simulink model "case8"  (R2024b)
settings: Solver=FixedStepAuto  StartTime=0  StopTime=1  FixedStep=1e-7  RelTol=1e-3
values from neighbouring files (symbols this model uses):
  SG_D_1_D = 0.01056    [IEEE9_case_parameters.m]    (also in case1_parameters.m; case2_parameters.m; case3_parameters.m; case4_parameters.m)
  SG_D_1_EnableSaturation = 0    [IEEE9_case_parameters.m]    (also in case1_parameters.m; case2_parameters.m; case3_parameters.m; case4_parameters.m)
  SG_D_1_f0 = 60    [IEEE9_case_parameters.m]    (also in case1_parameters.m; case2_parameters.m; case3_parameters.m; case4_parameters.m)
  SG_D_1_H = 7.5    [IEEE9_case_parameters.m]    (also in case1_parameters.m; case2_parameters.m; case3_parameters.m; case4_parameters.m)
  SG_D_1_K_A = 20    [IEEE9_case_parameters.m]    (also in case1_parameters.m; case2_parameters.m; case3_parameters.m; case4_parameters.m)
  SG_D_1_K_E = 1.000000e+1    (= 10)    [IEEE9_case_parameters.m]    (also in case1_parameters.m; case2_parameters.m; case3_parameters.m; case4_parameters.m)
  SG_D_1_K_F = 2.363    [IEEE9_case_parameters.m]    (also in case1_parameters.m; case2_parameters.m; case3_parameters.m; case4_parameters.m)
  SG_D_1_K_s = 0.5    [IEEE9_case_parameters.m]    (also in case1_parameters.m = 5; case2_parameters.m = 5; case3_parameters.m = 5; case4_parameters.m = 5)
  SG_D_1_R_a = 0.001088    [IEEE9_case_parameters.m]    (also in case1_parameters.m; case2_parameters.m; case3_parameters.m; case4_parameters.m)
  SG_D_1_S_A = 1    [IEEE9_case_parameters.m]    (also in case1_parameters.m; case2_parameters.m; case3_parameters.m; case4_parameters.m)
  SG_D_1_S_B = 0.103    [IEEE9_case_parameters.m]    (also in case1_parameters.m; case2_parameters.m; case3_parameters.m; case4_parameters.m)
  SG_D_1_S_N = 10.659857    [IEEE9_case_parameters.m]    (also in case1_parameters.m; case2_parameters.m; case3_parameters.m; case4_parameters.m)
  SG_D_1_SpeedPara = 200    [IEEE9_case_parameters.m]    (also in case1_parameters.m; case2_parameters.m; case3_parameters.m; case4_parameters.m)
  SG_D_1_T_0 = 0.720173    [IEEE9_case_parameters.m]    (also in case1_parameters.m = 0.755522; case2_parameters.m = 0.808931; case3_parameters.m = 0.869402; case4_parameters.m = 0.729316)
  SG_D_1_T_1 = 0.3    [IEEE9_case_parameters.m]    (also in case1_parameters.m; case2_parameters.m; case3_parameters.m; case4_parameters.m)
  SG_D_1_T_2 = 0.05    [IEEE9_case_parameters.m]    (also in case1_parameters.m; case2_parameters.m; case3_parameters.m; case4_parameters.m)
  SG_D_1_T_3 = 0.02    [IEEE9_case_parameters.m]    (also in case1_parameters.m; case2_parameters.m; case3_parameters.m; case4_parameters.m)
  SG_D_1_T_4 = 0.005    [IEEE9_case_parameters.m]    (also in case1_parameters.m; case2_parameters.m; case3_parameters.m; case4_parameters.m)
  SG_D_1_T_A = 0.02    [IEEE9_case_parameters.m]    (also in case1_parameters.m; case2_parameters.m; case3_parameters.m; case4_parameters.m)
  SG_D_1_T_dd = 8.000000e+0    (= 8)    [IEEE9_case_parameters.m]    (also in case1_parameters.m; case2_parameters.m; case3_parameters.m; case4_parameters.m)
  SG_D_1_T_ddd = 0.04    [IEEE9_case_parameters.m]    (also in case1_parameters.m; case2_parameters.m; case3_parameters.m; case4_parameters.m)
  SG_D_1_T_E = 0.314    [IEEE9_case_parameters.m]    (also in case1_parameters.m; case2_parameters.m; case3_parameters.m; case4_parameters.m)
  SG_D_1_T_F = 0.35    [IEEE9_case_parameters.m]    (also in case1_parameters.m; case2_parameters.m; case3_parameters.m; case4_parameters.m)
  SG_D_1_T_qd = 0.8    [IEEE9_case_parameters.m]    (also in case1_parameters.m; case2_parameters.m; case3_parameters.m; case4_parameters.m)
  SG_D_1_T_qdd = 0.02    [IEEE9_case_parameters.m]    (also in case1_parameters.m; case2_parameters.m; case3_parameters.m; case4_parameters.m)
  SG_D_1_T_speed = 0.1    [IEEE9_case_parameters.m]    (also in case1_parameters.m = 200; case2_parameters.m = 200; case3_parameters.m = 200; case4_parameters.m = 200)
  SG_D_1_T_w = 0.5    [IEEE9_case_parameters.m]    (also in case1_parameters.m; case2_parameters.m; case3_parameters.m; case4_parameters.m)
  SG_D_1_V_ref = 1.990276    [IEEE9_case_parameters.m]    (also in case1_parameters.m = 2.042296; case2_parameters.m = 2.051388; case3_parameters.m = 2.089584; case4_parameters.m = 2.01845)
  SG_D_1_w_ref = 376.991118    [IEEE9_case_parameters.m]    (also in case1_parameters.m; case2_parameters.m; case3_parameters.m; case4_parameters.m)
  SG_D_1_wb = 6.000000e+1    (= 60)    [IEEE9_case_parameters.m]    (also in case1_parameters.m; case2_parameters.m; case3_parameters.m; case4_parameters.m)
  SG_D_1_x_d = 1.9    [IEEE9_case_parameters.m]    (also in case1_parameters.m; case2_parameters.m; case3_parameters.m; case4_parameters.m)
  SG_D_1_x_dd = 0.302    [IEEE9_case_parameters.m]    (also in case1_parameters.m; case2_parameters.m; case3_parameters.m; case4_parameters.m)
  SG_D_1_x_ddd = 0.204    [IEEE9_case_parameters.m]    (also in case1_parameters.m; case2_parameters.m; case3_parameters.m; case4_parameters.m)
  SG_D_1_x_l = 0.05    [IEEE9_case_parameters.m]    (also in case1_parameters.m; case2_parameters.m; case3_parameters.m; case4_parameters.m)
  SG_D_1_x_q = 1.3    [IEEE9_case_parameters.m]    (also in case1_parameters.m; case2_parameters.m; case3_parameters.m; case4_parameters.m)
  SG_D_1_x_qd = 0.5    [IEEE9_case_parameters.m]    (also in case1_parameters.m; case2_parameters.m; case3_parameters.m; case4_parameters.m)
  SG_D_1_x_qdd = 0.3    [IEEE9_case_parameters.m]    (also in case1_parameters.m; case2_parameters.m; case3_parameters.m; case4_parameters.m)
  SG_D_2_D = 0.02    [IEEE9_case_parameters.m]    (also in case1_parameters.m; case2_parameters.m; case3_parameters.m; case4_parameters.m)
  SG_D_2_EnableSaturation = 0    [IEEE9_case_parameters.m]    (also in case1_parameters.m; case2_parameters.m; case3_parameters.m; case4_parameters.m)
  SG_D_2_f0 = 60    [IEEE9_case_parameters.m]    (also in case1_parameters.m; case2_parameters.m; case3_parameters.m; case4_parameters.m)
  SG_D_2_H = 8.000000e+0    (= 8)    [IEEE9_case_parameters.m]    (also in case1_parameters.m; case2_parameters.m; case3_parameters.m; case4_parameters.m)
  SG_D_2_K_A = 20    [IEEE9_case_parameters.m]    (also in case1_parameters.m; case2_parameters.m; case3_parameters.m; case4_parameters.m)
  SG_D_2_K_E = 1.000000e+1    (= 10)    [IEEE9_case_parameters.m]    (also in case1_parameters.m; case2_parameters.m; case3_parameters.m; case4_parameters.m)
  SG_D_2_K_F = 2.363    [IEEE9_case_parameters.m]    (also in case1_parameters.m; case2_parameters.m; case3_parameters.m; case4_parameters.m)
  SG_D_2_K_s = 0.5    [IEEE9_case_parameters.m]    (also in case1_parameters.m = 4; case2_parameters.m = 4; case3_parameters.m = 4; case4_parameters.m = 4)
  SG_D_2_R_a = 0.001088    [IEEE9_case_parameters.m]    (also in case1_parameters.m; case2_parameters.m; case3_parameters.m; case4_parameters.m)
  SG_D_2_S_A = 1    [IEEE9_case_parameters.m]    (also in case1_parameters.m; case2_parameters.m; case3_parameters.m; case4_parameters.m)
  SG_D_2_S_B = 0.103    [IEEE9_case_parameters.m]    (also in case1_parameters.m; case2_parameters.m; case3_parameters.m; case4_parameters.m)
  SG_D_2_S_N = 10.659857    [IEEE9_case_parameters.m]    (also in case1_parameters.m; case2_parameters.m; case3_parameters.m; case4_parameters.m)
  SG_D_2_SpeedPara = 200    [IEEE9_case_parameters.m]    (also in case1_parameters.m; case2_parameters.m; case3_parameters.m; case4_parameters.m)
  SG_D_2_T_0 = 1.632913    [IEEE9_case_parameters.m]    (also in case1_parameters.m = 1.632925; case2_parameters.m = 1.632915; case3_parameters.m = 1.632914; case4_parameters.m = 1.632927)
  SG_D_2_T_1 = 0.2    [IEEE9_case_parameters.m]    (also in case1_parameters.m; case2_parameters.m; case3_parameters.m; case4_parameters.m)
  SG_D_2_T_2 = 0.05    [IEEE9_case_parameters.m]    (also in case1_parameters.m; case2_parameters.m; case3_parameters.m; case4_parameters.m)
  SG_D_2_T_3 = 0.02    [IEEE9_case_parameters.m]    (also in case1_parameters.m; case2_parameters.m; case3_parameters.m; case4_parameters.m)
  SG_D_2_T_4 = 0.005    [IEEE9_case_parameters.m]    (also in case1_parameters.m; case2_parameters.m; case3_parameters.m; case4_parameters.m)
  SG_D_2_T_A = 0.02    [IEEE9_case_parameters.m]    (also in case1_parameters.m; case2_parameters.m; case3_parameters.m; case4_parameters.m)
  SG_D_2_T_dd = 7.9    [IEEE9_case_parameters.m]    (also in case1_parameters.m; case2_parameters.m; case3_parameters.m; case4_parameters.m)
  SG_D_2_T_ddd = 0.04    [IEEE9_case_parameters.m]    (also in case1_parameters.m; case2_parameters.m; case3_parameters.m; case4_parameters.m)
  SG_D_2_T_E = 0.314    [IEEE9_case_parameters.m]    (also in case1_parameters.m; case2_parameters.m; case3_parameters.m; case4_parameters.m)
  SG_D_2_T_F = 0.35    [IEEE9_case_parameters.m]    (also in case1_parameters.m; case2_parameters.m; case3_parameters.m; case4_parameters.m)
  SG_D_2_T_qd = 0.8    [IEEE9_case_parameters.m]    (also in case1_parameters.m; case2_parameters.m; case3_parameters.m; case4_parameters.m)
  SG_D_2_T_qdd = 0.015    [IEEE9_case_parameters.m]    (also in case1_parameters.m; case2_parameters.m; case3_parameters.m; case4_parameters.m)
  SG_D_2_T_speed = 0.1    [IEEE9_case_parameters.m]    (also in case1_parameters.m = 150; case2_parameters.m = 150; case3_parameters.m = 150; case4_parameters.m = 150)
  SG_D_2_T_w = 0.35    [IEEE9_case_parameters.m]    (also in case1_parameters.m; case2_parameters.m; case3_parameters.m; case4_parameters.m)
  SG_D_2_V_ref = 2.58547    [IEEE9_case_parameters.m]    (also in case1_parameters.m = 2.597896; case2_parameters.m = 2.587136; case3_parameters.m = 2.586042; case4_parameters.m = 2.599679)
  SG_D_2_w_ref = 376.991118    [IEEE9_case_parameters.m]    (also in case1_parameters.m; case2_parameters.m; case3_parameters.m; case4_parameters.m)
  SG_D_2_wb = 6.000000e+1    (= 60)    [IEEE9_case_parameters.m]    (also in case1_parameters.m; case2_parameters.m; case3_parameters.m; case4_parameters.m)
  SG_D_2_x_d = 1.8    [IEEE9_case_parameters.m]    (also in case1_parameters.m; case2_parameters.m; case3_parameters.m; case4_parameters.m)
  SG_D_2_x_dd = 0.302    [IEEE9_case_parameters.m]    (also in case1_parameters.m; case2_parameters.m; case3_parameters.m; case4_parameters.m)
  SG_D_2_x_ddd = 0.204    [IEEE9_case_parameters.m]    (also in case1_parameters.m; case2_parameters.m; case3_parameters.m; case4_parameters.m)
  SG_D_2_x_l = 0.05    [IEEE9_case_parameters.m]    (also in case1_parameters.m; case2_parameters.m; case3_parameters.m; case4_parameters.m)
  SG_D_2_x_q = 1.25    [IEEE9_case_parameters.m]    (also in case1_parameters.m; case2_parameters.m; case3_parameters.m; case4_parameters.m)
  SG_D_2_x_qd = 0.5    [IEEE9_case_parameters.m]    (also in case1_parameters.m; case2_parameters.m; case3_parameters.m; case4_parameters.m)
  SG_D_2_x_qdd = 0.3    [IEEE9_case_parameters.m]    (also in case1_parameters.m; case2_parameters.m; case3_parameters.m; case4_parameters.m)
  SG_D_3_D = 0.02    [IEEE9_case_parameters.m]    (also in case1_parameters.m; case2_parameters.m; case3_parameters.m; case4_parameters.m)
  SG_D_3_EnableSaturation = 0    [IEEE9_case_parameters.m]    (also in case1_parameters.m; case2_parameters.m; case3_parameters.m; case4_parameters.m)
  SG_D_3_f0 = 60    [IEEE9_case_parameters.m]    (also in case1_parameters.m; case2_parameters.m; case3_parameters.m; case4_parameters.m)
  SG_D_3_H = 7.7    [IEEE9_case_parameters.m]    (also in case1_parameters.m; case2_parameters.m; case3_parameters.m; case4_parameters.m)
  SG_D_3_K_A = 20    [IEEE9_case_parameters.m]    (also in case1_parameters.m; case2_parameters.m; case3_parameters.m; case4_parameters.m)
  SG_D_3_K_E = 1.000000e+1    (= 10)    [IEEE9_case_parameters.m]    (also in case1_parameters.m; case2_parameters.m; case3_parameters.m; case4_parameters.m)
  SG_D_3_K_F = 2.363    [IEEE9_case_parameters.m]    (also in case1_parameters.m; case2_parameters.m; case3_parameters.m; case4_parameters.m)
  SG_D_3_K_s = 0.2    [IEEE9_case_parameters.m]    (also in case1_parameters.m = 2; case2_parameters.m = 2; case3_parameters.m = 2; case4_parameters.m = 2)
  SG_D_3_R_a = 0.001088    [IEEE9_case_parameters.m]    (also in case1_parameters.m; case2_parameters.m; case3_parameters.m; case4_parameters.m)
  SG_D_3_S_A = 1    [IEEE9_case_parameters.m]    (also in case1_parameters.m; case2_parameters.m; case3_parameters.m; case4_parameters.m)
  SG_D_3_S_B = 0.103    [IEEE9_case_parameters.m]    (also in case1_parameters.m; case2_parameters.m; case3_parameters.m; case4_parameters.m)
  SG_D_3_S_N = 10.659857    [IEEE9_case_parameters.m]    (also in case1_parameters.m; case2_parameters.m; case3_parameters.m; case4_parameters.m)
  SG_D_3_SpeedPara = 200    [IEEE9_case_parameters.m]    (also in case1_parameters.m; case2_parameters.m; case3_parameters.m; case4_parameters.m)
  SG_D_3_T_0 = 0.850788    [IEEE9_case_parameters.m]    (also in case1_parameters.m = 0.850786; case2_parameters.m = 0.850787; case3_parameters.m; case4_parameters.m = 0.850786)
  SG_D_3_T_1 = 0.2    [IEEE9_case_parameters.m]    (also in case1_parameters.m; case2_parameters.m; case3_parameters.m; case4_parameters.m)
  SG_D_3_T_2 = 0.05    [IEEE9_case_parameters.m]    (also in case1_parameters.m; case2_parameters.m; case3_parameters.m; case4_parameters.m)
  SG_D_3_T_3 = 0.02    [IEEE9_case_parameters.m]    (also in case1_parameters.m; case2_parameters.m; case3_parameters.m; case4_parameters.m)
  SG_D_3_T_4 = 0.005    [IEEE9_case_parameters.m]    (also in case1_parameters.m; case2_parameters.m; case3_parameters.m; case4_parameters.m)
  SG_D_3_T_A = 0.02    [IEEE9_case_parameters.m]    (also in case1_parameters.m; case2_parameters.m; case3_parameters.m; case4_parameters.m)
  SG_D_3_T_dd = 8.1    [IEEE9_case_parameters.m]    (also in case1_parameters.m; case2_parameters.m; case3_parameters.m; case4_parameters.m)
  SG_D_3_T_ddd = 0.04    [IEEE9_case_parameters.m]    (also in case1_parameters.m; case2_parameters.m; case3_parameters.m; case4_parameters.m)
  SG_D_3_T_E = 0.314    [IEEE9_case_parameters.m]    (also in case1_parameters.m; case2_parameters.m; case3_parameters.m; case4_parameters.m)
  SG_D_3_T_F = 0.35    [IEEE9_case_parameters.m]    (also in case1_parameters.m; case2_parameters.m; case3_parameters.m; case4_parameters.m)
  SG_D_3_T_qd = 0.8    [IEEE9_case_parameters.m]    (also in case1_parameters.m; case2_parameters.m; case3_parameters.m; case4_parameters.m)
  SG_D_3_T_qdd = 0.015    [IEEE9_case_parameters.m]    (also in case1_parameters.m; case2_parameters.m; case3_parameters.m; case4_parameters.m)
  SG_D_3_T_speed = 0.1    [IEEE9_case_parameters.m]    (also in case1_parameters.m = 180; case2_parameters.m = 180; case3_parameters.m = 180; case4_parameters.m = 180)
  SG_D_3_T_w = 0.4    [IEEE9_case_parameters.m]    (also in case1_parameters.m; case2_parameters.m; case3_parameters.m; case4_parameters.m)
  SG_D_3_V_ref = 1.892727    [IEEE9_case_parameters.m]    (also in case1_parameters.m = 1.906439; case2_parameters.m = 1.895535; case3_parameters.m = 1.892105; case4_parameters.m = 1.906598)
  SG_D_3_w_ref = 376.991118    [IEEE9_case_parameters.m]    (also in case1_parameters.m; case2_parameters.m; case3_parameters.m; case4_parameters.m)
  SG_D_3_wb = 6.000000e+1    (= 60)    [IEEE9_case_parameters.m]    (also in case1_parameters.m; case2_parameters.m; case3_parameters.m; case4_parameters.m)
  SG_D_3_x_d = 1.85    [IEEE9_case_parameters.m]    (also in case1_parameters.m; case2_parameters.m; case3_parameters.m; case4_parameters.m)
  SG_D_3_x_dd = 0.302    [IEEE9_case_parameters.m]    (also in case1_parameters.m; case2_parameters.m; case3_parameters.m; case4_parameters.m)
  SG_D_3_x_ddd = 0.204    [IEEE9_case_parameters.m]    (also in case1_parameters.m; case2_parameters.m; case3_parameters.m; case4_parameters.m)
  SG_D_3_x_l = 0.05    [IEEE9_case_parameters.m]    (also in case1_parameters.m; case2_parameters.m; case3_parameters.m; case4_parameters.m)
  SG_D_3_x_q = 1.2    [IEEE9_case_parameters.m]    (also in case1_parameters.m; case2_parameters.m; case3_parameters.m; case4_parameters.m)
  SG_D_3_x_qd = 0.5    [IEEE9_case_parameters.m]    (also in case1_parameters.m; case2_parameters.m; case3_parameters.m; case4_parameters.m)
  SG_D_3_x_qdd = 0.3    [IEEE9_case_parameters.m]    (also in case1_parameters.m; case2_parameters.m; case3_parameters.m; case4_parameters.m)
(part 7 of 12)

== system case8/SG_D_2/T_e_SG_D_2_block ==
  note: T_e_SG_D_2 in case8
      | $-\frac{\psi _{d,\mathrm{SG},D,2}\,\left(\psi _{q,\mathrm{SG},D,2}+\frac{\psi _{\mathrm{gq},\mathrm{SG},D,2}\,\left(x_{l}-x_{\mathrm{qdd}}\right)}{x_{l}-x_{\mathrm{qd}}}+\frac{\psi _{\mathrm{kq},\mathrm{SG},D,2}\,\left(x_{\mathrm{qd}}-x_{\mathrm{qdd}}\right)}{x_{l}-x_{\mathrm{qd}}}\right)}{x_{\mathrm{qdd}}}-\frac{\psi _{q,\mathrm{SG},D,2}\,\left(\frac{\psi _{\mathrm{1d},\mathrm{SG},D,2}\,\left(x_{\mathrm{dd}}-x_{\mathrm{ddd}}\right)}{x_{\mathrm{dd}}-x_{l}}-\psi _{d,\mathrm{SG},D,2}+\frac{\psi _{\mathrm{fd},\mathrm{SG},D,2}\,\left(x_{\mathrm{ddd}}-x_{l}\right)}{x_{\mathrm{dd}}-x_{l}}\right)}{x_{\mathrm{ddd}}}$
      | Automatically generated on 2025-10-31 19:30:01 .
  State_psi_d_SG_D_2_f5fd7 : Inport
  State_psi_gq_SG_D_2_6b895 : Inport  Port=2
  State_psi_kq_SG_D_2_20085 : Inport  Port=3
  State_psi_q_SG_D_2_d1f35 : Inport  Port=4
  State_psi_q_SG_D_2_dcfde : Inport  Port=5
  State_psi_1d_SG_D_2_b2612 : Inport  Port=6
  State_psi_d_SG_D_2_0c163 : Inport  Port=7
  State_psi_fd_SG_D_2_89a99 : Inport  Port=8
  Add_136e4 : Sum
  Add_53914 : Sum
  Add_61d82 : Sum
  Add_773d3 : Sum
  Add_83d4e : Sum
  Add_d6d3e : Sum
  Constant_-1_009c4 : Constant  Value=-1
  Constant_-1_892f0 : Constant  Value=-1
  Constant_-1_8f9af : Constant  Value=-1
  Constant_-1_ac596 : Constant  Value=-1
  Constant_-1_f984b : Constant  Value=-1
  Constant_x_dd_539a3 : Constant  Value=x_dd
  Constant_x_dd_5f008 : Constant  Value=x_dd
  Constant_x_dd_6f2fd : Constant  Value=x_dd
  Constant_x_ddd_43beb : Constant  Value=x_ddd
  Constant_x_ddd_5974d : Constant  Value=x_ddd
  Constant_x_ddd_df5c6 : Constant  Value=x_ddd
  Constant_x_l_1b4ed : Constant  Value=x_l
  Constant_x_l_21d9c : Constant  Value=x_l
  Constant_x_l_82116 : Constant  Value=x_l
  Constant_x_l_9e257 : Constant  Value=x_l
  Constant_x_l_ccf6e : Constant  Value=x_l
  Constant_x_l_da74a : Constant  Value=x_l
  Constant_x_qd_305c8 : Constant  Value=x_qd
  Constant_x_qd_c568d : Constant  Value=x_qd
  Constant_x_qd_e5ab0 : Constant  Value=x_qd
  Constant_x_qdd_23062 : Constant  Value=x_qdd
  Constant_x_qdd_642dc : Constant  Value=x_qdd
  Constant_x_qdd_bb207 : Constant  Value=x_qdd
  Divide_1324e : Product  Inputs=*/
  Divide_1c984 : Product  Inputs=*/
  Divide_4d64c : Product  Inputs=*/
  Divide_4f496 : Product  Inputs=*/
  Divide_cc898 : Product  Inputs=*/
  Divide_d40a1 : Product  Inputs=*/
  Product_2226e : Product
  Product_299f3 : Product
  Product_47b76 : Product
  Product_50440 : Product
  Product_582c1 : Product
  Product_6692e : Product
  Product_6acbc : Product
  Product_6f7a7 : Product
  Product_75582 : Product
  Product_78bca : Product
  Product_7dbfb : Product
  Subtract_00826 : Sum  Inputs=+-
  Subtract_1342e : Sum  Inputs=+-
  Subtract_3f03d : Sum  Inputs=+-
  Subtract_5a401 : Sum  Inputs=+-
  Subtract_9aa6a : Sum  Inputs=+-
  Subtract_c14d6 : Sum  Inputs=+-
  Subtract_caa32 : Sum  Inputs=+-
  Blockout_T_e_SG_D_2_37eed : Outport
  wires:
  Constant_-1_892f0/1 -> Product_299f3/1
  Divide_1c984/1 -> Subtract_3f03d/1
  Constant_-1_ac596/1 -> Product_2226e/1
  Constant_x_l_da74a/1 -> Product_2226e/2
  Constant_x_qd_e5ab0/1 -> Subtract_caa32/1
  Product_78bca/1 -> Divide_1c984/1
  Product_2226e/1 -> Add_773d3/1
  Divide_cc898/1 -> Subtract_c14d6/2
  Constant_x_qdd_642dc/1 -> Subtract_caa32/2
  Constant_x_qdd_23062/1 -> Divide_4f496/2
  Constant_x_ddd_5974d/1 -> Subtract_9aa6a/2
  Constant_x_qdd_bb207/1 -> Add_773d3/2
  Constant_x_l_82116/1 -> Product_299f3/2
  Constant_-1_009c4/1 -> Product_75582/1
  Constant_x_l_ccf6e/1 -> Product_75582/2
  Constant_-1_8f9af/1 -> Product_6acbc/1
  State_psi_1d_SG_D_2_b2612/1 -> Product_6acbc/2
  Constant_x_dd_5f008/1 -> Subtract_9aa6a/1
  Divide_4d64c/1 -> Subtract_3f03d/2
  State_psi_gq_SG_D_2_6b895/1 -> Product_78bca/1
  Add_773d3/1 -> Product_78bca/2
  Subtract_3f03d/1 -> Add_136e4/1
  Constant_x_dd_539a3/1 -> Subtract_00826/1
  Product_299f3/1 -> Add_83d4e/1
  Product_582c1/1 -> Product_50440/1
  Constant_x_qd_305c8/1 -> Add_83d4e/2
  State_psi_kq_SG_D_2_20085/1 -> Product_6692e/1
  Subtract_caa32/1 -> Product_6692e/2
  Product_75582/1 -> Add_61d82/1
  State_psi_q_SG_D_2_dcfde/1 -> Product_47b76/1
  Constant_x_qd_c568d/1 -> Add_61d82/2
  Product_6acbc/1 -> Product_6f7a7/1
  Divide_1324e/1 -> Add_53914/2
  Subtract_9aa6a/1 -> Product_6f7a7/2
  Constant_x_l_1b4ed/1 -> Subtract_00826/2
  Constant_x_ddd_df5c6/1 -> Subtract_5a401/1
  Constant_x_dd_6f2fd/1 -> Subtract_1342e/1
  Constant_x_l_21d9c/1 -> Subtract_5a401/2
  Add_53914/1 -> Blockout_T_e_SG_D_2_37eed/1
  Add_83d4e/1 -> Divide_1c984/2
  Product_6692e/1 -> Divide_4d64c/1
  Product_50440/1 -> Divide_4f496/1
  State_psi_d_SG_D_2_f5fd7/1 -> Product_582c1/2
  Add_61d82/1 -> Divide_4d64c/2
  Product_6f7a7/1 -> Divide_d40a1/1
  Subtract_00826/1 -> Divide_d40a1/2
  Constant_x_l_9e257/1 -> Subtract_1342e/2
  State_psi_fd_SG_D_2_89a99/1 -> Product_7dbfb/1
  Constant_x_ddd_43beb/1 -> Divide_1324e/2
  Product_47b76/1 -> Divide_1324e/1
  Subtract_5a401/1 -> Product_7dbfb/2
  Divide_d40a1/1 -> Add_d6d3e/1
  State_psi_d_SG_D_2_0c163/1 -> Add_d6d3e/2
  Add_d6d3e/1 -> Subtract_c14d6/1
  Product_7dbfb/1 -> Divide_cc898/1
  Subtract_1342e/1 -> Divide_cc898/2
  Constant_-1_f984b/1 -> Product_582c1/1
  State_psi_q_SG_D_2_d1f35/1 -> Add_136e4/2
  Add_136e4/1 -> Product_50440/2
  Subtract_c14d6/1 -> Product_47b76/2
  Divide_4f496/1 -> Add_53914/1

== system case8/SG_D_2/d_E_fd_SG_D_2_block ==
  note: d_E_fd_SG_D_2 in case8
      | $\frac{V_{f,\mathrm{SG},D,2}-E_{\mathrm{fd},\mathrm{SG},D,2}\,K_{E}}{T_{E}}$
      | Automatically generated on 2025-10-31 19:29:56 .
  State_E_fd_SG_D_2_423a9 : Inport
  State_V_f_SG_D_2_b3f2e : Inport  Port=2
  Add_25b17 : Sum
  Constant_-1_61e25 : Constant  Value=-1
  Constant_K_E_4608d : Constant  Value=K_E
  Constant_T_E_94d73 : Constant  Value=T_E
  Divide_83db9 : Product  Inputs=*/
  Product_0c2eb : Product
  Product_b81d0 : Product
  Blockout_d_E_fd_SG_D_2_a4411 : Outport
  wires:
  Constant_-1_61e25/1 -> Product_0c2eb/1
  State_E_fd_SG_D_2_423a9/1 -> Product_0c2eb/2
  Product_0c2eb/1 -> Product_b81d0/1
  Constant_K_E_4608d/1 -> Product_b81d0/2
  Product_b81d0/1 -> Add_25b17/1
  Constant_T_E_94d73/1 -> Divide_83db9/2
  State_V_f_SG_D_2_b3f2e/1 -> Add_25b17/2
  Add_25b17/1 -> Divide_83db9/1
  Divide_83db9/1 -> Blockout_d_E_fd_SG_D_2_a4411/1

== system case8/SG_D_2/d_Px_1_SG_D_2_block ==
  note: d_Px_1_SG_D_2 in case8
      | $\frac{w_{\mathrm{SG},D,2}-2\,\pi \,f_{0}}{T_{w}}-\frac{\mathrm{Px}_{1,\mathrm{SG},D,2}}{T_{w}}$
      | Automatically generated on 2025-10-31 19:29:57 .
  State_Px_1_SG_D_2_1fdac : Inport
  State_w_SG_D_2_e8896 : Inport  Port=2
  Add_4c732 : Sum
  Add_5193f : Sum
  Constant_-1_69875 : Constant  Value=-1
  Constant_-2.0_497bd : Constant  Value=-2.0
  Constant_T_w_ca876 : Constant  Value=T_w
  Constant_T_w_db7d6 : Constant  Value=T_w
  Constant_f0_826e2 : Constant  Value=f0
  Constant_pi_6538e : Constant  Value=pi
  Divide_c5870 : Product  Inputs=*/
  Divide_dfdb0 : Product  Inputs=*/
  Product_c48f8 : Product
  Product_d32d8 : Product
  Product_f4819 : Product
  Blockout_d_Px_1_SG_D_2_3d98f : Outport
  wires:
  Constant_-2.0_497bd/1 -> Product_d32d8/1
  State_w_SG_D_2_e8896/1 -> Add_5193f/2
  Constant_pi_6538e/1 -> Product_d32d8/2
  Product_d32d8/1 -> Product_c48f8/1
  Constant_f0_826e2/1 -> Product_c48f8/2
  Constant_-1_69875/1 -> Product_f4819/1
  State_Px_1_SG_D_2_1fdac/1 -> Product_f4819/2
  Product_c48f8/1 -> Add_5193f/1
  Product_f4819/1 -> Divide_dfdb0/1
  Constant_T_w_ca876/1 -> Divide_dfdb0/2
  Add_5193f/1 -> Divide_c5870/1
  Constant_T_w_db7d6/1 -> Divide_c5870/2
  Divide_dfdb0/1 -> Add_4c732/1
  Divide_c5870/1 -> Add_4c732/2
  Add_4c732/1 -> Blockout_d_Px_1_SG_D_2_3d98f/1

== system case8/SG_D_2/d_Px_2_SG_D_2_block ==
  note: d_Px_2_SG_D_2 in case8
      | $\frac{\mathrm{Px}_{1,\mathrm{SG},D,2}-T_{2}\,\left(\frac{\mathrm{Px}_{1,\mathrm{SG},D,2}}{T_{w}}-\frac{w_{\mathrm{SG},D,2}-2\,\pi \,f_{0}}{T_{w}}\right)}{T_{1}}-\frac{\mathrm{Px}_{2,\mathrm{SG},D,2}}{T_{1}}$
      | Automatically generated on 2025-10-31 19:29:57 .
  State_Px_2_SG_D_2_8f0fc : Inport
  State_Px_1_SG_D_2_d6347 : Inport  Port=2
  State_Px_1_SG_D_2_2790d : Inport  Port=3
  State_w_SG_D_2_770a4 : Inport  Port=4
  Add_36fde : Sum
  Add_9a15f : Sum
  Add_aade0 : Sum
  Add_f8e8c : Sum
  Constant_-1_a4b81 : Constant  Value=-1
  Constant_-1_c1136 : Constant  Value=-1
  Constant_-2.0_37c36 : Constant  Value=-2.0
  Constant_T_1_313c9 : Constant  Value=T_1
  Constant_T_1_99444 : Constant  Value=T_1
  Constant_T_2_214de : Constant  Value=T_2
  Constant_T_w_0eda0 : Constant  Value=T_w
  Constant_T_w_a5a3c : Constant  Value=T_w
  Constant_f0_de17b : Constant  Value=f0
  Constant_pi_860d9 : Constant  Value=pi
  Divide_48f92 : Product  Inputs=*/
  Divide_8705a : Product  Inputs=*/
  Divide_c60fc : Product  Inputs=*/
  Divide_fd14b : Product  Inputs=*/
  Product_30601 : Product
  Product_5dbb0 : Product
  Product_6c663 : Product
  Product_bcc78 : Product
  Product_e83f9 : Product
  Blockout_d_Px_2_SG_D_2_834a7 : Outport
  wires:
  Constant_-1_a4b81/1 -> Product_bcc78/1
  Constant_-2.0_37c36/1 -> Product_5dbb0/1
  Product_e83f9/1 -> Add_f8e8c/2
  State_w_SG_D_2_770a4/1 -> Add_aade0/2
  Constant_pi_860d9/1 -> Product_5dbb0/2
  Product_5dbb0/1 -> Product_6c663/1
  State_Px_1_SG_D_2_2790d/1 -> Product_30601/2
  Constant_f0_de17b/1 -> Product_6c663/2
  State_Px_2_SG_D_2_8f0fc/1 -> Product_bcc78/2
  Constant_-1_c1136/1 -> Product_30601/1
  Product_6c663/1 -> Add_aade0/1
  Product_30601/1 -> Divide_48f92/1
  Constant_T_w_a5a3c/1 -> Divide_48f92/2
  Add_aade0/1 -> Divide_fd14b/1
  Constant_T_w_0eda0/1 -> Divide_fd14b/2
  Divide_48f92/1 -> Add_9a15f/1
  Divide_fd14b/1 -> Add_9a15f/2
  Constant_T_2_214de/1 -> Product_e83f9/1
  Add_9a15f/1 -> Product_e83f9/2
  State_Px_1_SG_D_2_d6347/1 -> Add_f8e8c/1
  Product_bcc78/1 -> Divide_c60fc/1
  Constant_T_1_99444/1 -> Divide_c60fc/2
  Add_f8e8c/1 -> Divide_8705a/1
  Constant_T_1_313c9/1 -> Divide_8705a/2
  Divide_c60fc/1 -> Add_36fde/1
  Divide_8705a/1 -> Add_36fde/2
  Add_36fde/1 -> Blockout_d_Px_2_SG_D_2_834a7/1

== system case8/SG_D_2/d_Px_3_SG_D_2_block ==
  note: d_Px_3_SG_D_2 in case8
      | $\frac{\mathrm{Px}_{2,\mathrm{SG},D,2}+T_{4}\,\left(\frac{\mathrm{Px}_{1,\mathrm{SG},D,2}-T_{2}\,\left(\frac{\mathrm{Px}_{1,\mathrm{SG},D,2}}{T_{w}}-\frac{w_{\mathrm{SG},D,2}-2\,\pi \,f_{0}}{T_{w}}\right)}{T_{1}}-\frac{\mathrm{Px}_{2,\mathrm{SG},D,2}}{T_{1}}\right)}{T_{3}}-\frac{\mathrm{Px}_{3,\mathrm{SG},D,2}}{T_{3}}$
      | Automatically generated on 2025-10-31 19:29:58 .
  State_Px_3_SG_D_2_a00f9 : Inport
  State_Px_2_SG_D_2_e8830 : Inport  Port=2
  State_Px_2_SG_D_2_b92ad : Inport  Port=3
  State_Px_1_SG_D_2_7fb84 : Inport  Port=4
  State_Px_1_SG_D_2_3fef0 : Inport  Port=5
  State_w_SG_D_2_e0f2c : Inport  Port=6
  Add_3c5a4 : Sum
  Add_45cb1 : Sum
  Add_478fb : Sum
  Add_98fbb : Sum
  Add_c2473 : Sum
  Add_e28b8 : Sum
  Constant_-1_3360d : Constant  Value=-1
  Constant_-1_357f0 : Constant  Value=-1
  Constant_-1_d3ba9 : Constant  Value=-1
  Constant_-2.0_0c54b : Constant  Value=-2.0
  Constant_T_1_5ca23 : Constant  Value=T_1
  Constant_T_1_645ff : Constant  Value=T_1
  Constant_T_2_9f8bc : Constant  Value=T_2
  Constant_T_3_25afd : Constant  Value=T_3
  Constant_T_3_a1775 : Constant  Value=T_3
  Constant_T_4_97e42 : Constant  Value=T_4
  Constant_T_w_3102e : Constant  Value=T_w
  Constant_T_w_b16aa : Constant  Value=T_w
  Constant_f0_93310 : Constant  Value=f0
  Constant_pi_9ec7e : Constant  Value=pi
  Divide_03af6 : Product  Inputs=*/
  Divide_5d724 : Product  Inputs=*/
  Divide_70b54 : Product  Inputs=*/
  Divide_cf44f : Product  Inputs=*/
  Divide_d5d88 : Product  Inputs=*/
  Divide_fecd8 : Product  Inputs=*/
  Product_0c09d : Product
  Product_1e5b6 : Product
  Product_83b7e : Product
  Product_87485 : Product
  Product_905df : Product
  Product_be3e8 : Product
  Product_df649 : Product
  Blockout_d_Px_3_SG_D_2_f4998 : Outport
  wires:
  Constant_-2.0_0c54b/1 -> Product_87485/1
  State_w_SG_D_2_e0f2c/1 -> Add_3c5a4/2
  Add_c2473/1 -> Divide_cf44f/1
  Constant_pi_9ec7e/1 -> Product_87485/2
  Constant_-1_d3ba9/1 -> Product_be3e8/1
  Product_87485/1 -> Product_83b7e/1
  State_Px_2_SG_D_2_b92ad/1 -> Product_be3e8/2
  State_Px_1_SG_D_2_3fef0/1 -> Product_905df/2
  Divide_cf44f/1 -> Add_478fb/2
  Constant_f0_93310/1 -> Product_83b7e/2
  Constant_-1_357f0/1 -> Product_905df/1
  Product_83b7e/1 -> Add_3c5a4/1
  Product_905df/1 -> Divide_d5d88/1
  Constant_T_w_b16aa/1 -> Divide_d5d88/2
  Divide_70b54/1 -> Add_478fb/1
  Add_3c5a4/1 -> Divide_03af6/1
  Product_0c09d/1 -> Add_98fbb/2
  Constant_T_w_3102e/1 -> Divide_03af6/2
  Divide_d5d88/1 -> Add_45cb1/1
  State_Px_1_SG_D_2_7fb84/1 -> Add_98fbb/1
  Divide_03af6/1 -> Add_45cb1/2
  Constant_-1_3360d/1 -> Product_1e5b6/1
  Constant_T_2_9f8bc/1 -> Product_0c09d/1
  Add_45cb1/1 -> Product_0c09d/2
  Product_be3e8/1 -> Divide_fecd8/1
  Constant_T_1_645ff/1 -> Divide_fecd8/2
  Add_98fbb/1 -> Divide_5d724/1
  Constant_T_1_5ca23/1 -> Divide_5d724/2
  Divide_fecd8/1 -> Add_e28b8/1
  Divide_5d724/1 -> Add_e28b8/2
  Constant_T_4_97e42/1 -> Product_df649/1
  Add_e28b8/1 -> Product_df649/2
  State_Px_3_SG_D_2_a00f9/1 -> Product_1e5b6/2
  State_Px_2_SG_D_2_e8830/1 -> Add_c2473/1
  Product_df649/1 -> Add_c2473/2
  Product_1e5b6/1 -> Divide_70b54/1
  Constant_T_3_a1775/1 -> Divide_70b54/2
  Constant_T_3_25afd/1 -> Divide_cf44f/2
  Add_478fb/1 -> Blockout_d_Px_3_SG_D_2_f4998/1

== system case8/SG_D_2/d_R_f_SG_D_2_block ==
  note: d_R_f_SG_D_2 in case8
      | $-\frac{R_{f,\mathrm{SG},D,2}-\frac{E_{\mathrm{fd},\mathrm{SG},D,2}\,K_{F}}{T_{F}}}{T_{F}}$
      | Automatically generated on 2025-10-31 19:29:56 .
  State_E_fd_SG_D_2_59077 : Inport
  State_R_f_SG_D_2_76268 : Inport  Port=2
  Constant_K_F_8fb42 : Constant  Value=K_F
  Constant_T_F_492c7 : Constant  Value=T_F
  Constant_T_F_7a55d : Constant  Value=T_F
  Divide_1705c : Product  Inputs=*/
  Divide_c19ba : Product  Inputs=*/
  Product_2540e : Product
  Subtract_aa317 : Sum  Inputs=+-
  Blockout_d_R_f_SG_D_2_8501b : Outport
  wires:
  Constant_T_F_7a55d/1 -> Divide_1705c/2
  State_E_fd_SG_D_2_59077/1 -> Product_2540e/1
  Constant_K_F_8fb42/1 -> Product_2540e/2
  State_R_f_SG_D_2_76268/1 -> Subtract_aa317/2
  Product_2540e/1 -> Divide_1705c/1
  Divide_1705c/1 -> Subtract_aa317/1
  Constant_T_F_492c7/1 -> Divide_c19ba/2
  Subtract_aa317/1 -> Divide_c19ba/1
  Divide_c19ba/1 -> Blockout_d_R_f_SG_D_2_8501b/1

== system case8/SG_D_2/d_T_m_SG_D_2_block ==
  note: d_T_m_SG_D_2 in case8
      | $-\frac{T_{m,\mathrm{SG},D,2}-T_{0}+\frac{\mathrm{SpeedPara}\,\left(w_{\mathrm{SG},D,2}-w_{\mathrm{ref}}\right)}{2\,f_{0}\,\pi }}{T_{\mathrm{speed}}}$
      | Automatically generated on 2025-10-31 19:29:54 .
  State_w_SG_D_2_f6fcd : Inport
  State_T_m_SG_D_2_95b0e : Inport  Port=2
  Add_2317b : Sum
  Add_41ec9 : Sum
  Constant_-1_4ba95 : Constant  Value=-1
  Constant_2.0_25eb2 : Constant  Value=2.0
  Constant_SpeedPara_0fd14 : Constant  Value=SpeedPara
  Constant_T_0_72408 : Constant  Value=T_0
  Constant_T_speed_db217 : Constant  Value=T_speed
  Constant_f0_1dd2e : Constant  Value=f0
  Constant_pi_74fbc : Constant  Value=pi
  Constant_w_ref_3c240 : Constant  Value=w_ref
  Divide_b7933 : Product  Inputs=*/
  Divide_e5622 : Product  Inputs=*/
  Product_35d20 : Product
  Product_815ed : Product
  Product_d1949 : Product
  Product_f5924 : Product
  Subtract_c4e7f : Sum  Inputs=+-
  Blockout_d_T_m_SG_D_2_9d432 : Outport
  wires:
  Constant_pi_74fbc/1 -> Product_f5924/2
  Constant_-1_4ba95/1 -> Product_815ed/1
  Constant_w_ref_3c240/1 -> Add_2317b/2
  State_w_SG_D_2_f6fcd/1 -> Product_815ed/2
  Product_815ed/1 -> Add_2317b/1
  Add_41ec9/1 -> Subtract_c4e7f/1
  Add_2317b/1 -> Product_35d20/2
  Constant_2.0_25eb2/1 -> Product_f5924/1
  Constant_SpeedPara_0fd14/1 -> Product_35d20/1
  Product_f5924/1 -> Product_d1949/1
  Constant_f0_1dd2e/1 -> Product_d1949/2
  Product_35d20/1 -> Divide_b7933/1
  Product_d1949/1 -> Divide_b7933/2
  Divide_b7933/1 -> Add_41ec9/1
  Constant_T_0_72408/1 -> Add_41ec9/2
  State_T_m_SG_D_2_95b0e/1 -> Subtract_c4e7f/2
  Subtract_c4e7f/1 -> Divide_e5622/1
  Constant_T_speed_db217/1 -> Divide_e5622/2
  Divide_e5622/1 -> Blockout_d_T_m_SG_D_2_9d432/1

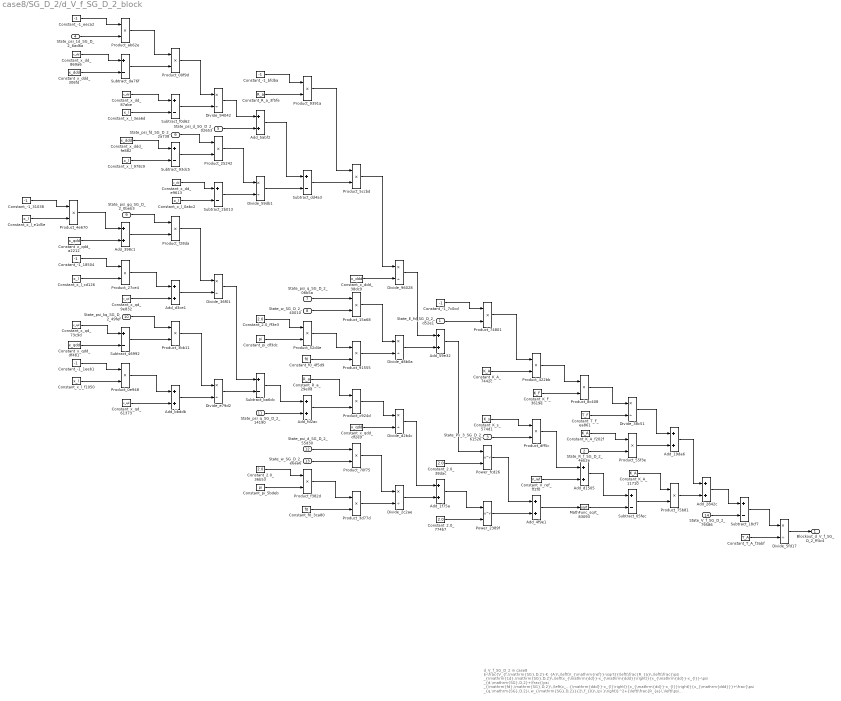
== system case8/SG_D_2/d_V_f_SG_D_2_block ==
  note: d_V_f_SG_D_2 in case8
      | $-\frac{V_{f,\mathrm{SG},D,2}-K_{A}\,\left(V_{\mathrm{ref}}-\sqrt{{\left(\frac{R_{a}\,\left(\frac{\psi _{\mathrm{1d},\mathrm{SG},D,2}\,\left(x_{\mathrm{dd}}-x_{\mathrm{ddd}}\right)}{x_{\mathrm{dd}}-x_{l}}-\psi _{d,\mathrm{SG},D,2}+\frac{\psi _{\mathrm{fd},\mathrm{SG},D,2}\,\left(x_{\mathrm{ddd}}-x_{l}\right)}{x_{\mathrm{dd}}-x_{l}}\right)}{x_{\mathrm{ddd}}}+\frac{\psi _{q,\mathrm{SG},D,2}\,w_{\mathrm{SG},D,2}}{2\,f_{0}\,\pi }\right)}^2+{\left(\frac{R_{a}\,\left(\psi _{q,\mathrm{SG},D,2}+\frac{\psi _{\mathrm{gq},\mathrm{SG},D,2}\,\left(x_{l}-x_{\mathrm{qdd}}\right)}{x_{l}-x_{\mathrm{qd}}}+\frac{\psi _{\mathrm{kq},\mathrm{SG},D,2}\,\left(x_{\mathrm{qd}}-x_{\mathrm{qdd}}\right)}{x_{l}-x_{\mathrm{qd}}}\right)}{x_{\mathrm{qdd}}}+\frac{\psi _{d,\mathrm{SG},D,2}\,w_{\mathrm{SG},D,2}}{2\,f_{0}\,\pi }\right)}^2}+K_{s}\,\mathrm{Px}_{3,\mathrm{SG},D,2}\right)-K_{A}\,R_{f,\mathrm{SG},D,2}+\frac{E_{\mathrm{fd},\mathrm{SG},D,2}\,K_{A}\,K_{F}}{T_{F}}}{T_{A}}$
      | Automatically generated on 2025-10-31 19:29:55 .
  State_E_fd_SG_D_2_d52e1 : Inport
  State_R_f_SG_D_2_4eb2e : Inport  Port=2
  State_Px_3_SG_D_2_61526 : Inport  Port=3
  State_psi_1d_SG_D_2_6ad6a : Inport  Port=4
  State_psi_d_SG_D_2_02653 : Inport  Port=5
  State_psi_fd_SG_D_2_2a738 : Inport  Port=6
  State_psi_q_SG_D_2_06b5a : Inport  Port=7
  State_w_SG_D_2_40010 : Inport  Port=8
  State_psi_gq_SG_D_2_0beb3 : Inport  Port=9
  State_psi_kq_SG_D_2_49fef : Inport  Port=10
  State_psi_q_SG_D_2_14190 : Inport  Port=11
  State_psi_d_SG_D_2_55d30 : Inport  Port=12
  State_w_SG_D_2_e6aa6 : Inport  Port=13
  State_V_f_SG_D_2_79586 : Inport  Port=14
  Add_19da6 : Sum
  Add_1f75a : Sum
  Add_2842c : Sum
  Add_398c1 : Sum
  Add_4f9e1 : Sum
  Add_59e32 : Sum
  Add_5abf2 : Sum
  Add_bbddb : Sum
  Add_d1505 : Sum
  Add_d3ce1 : Sum
  Add_fd2ac : Sum
  Constant_-1_18504 : Constant  Value=-1
  Constant_-1_1eeb1 : Constant  Value=-1
  Constant_-1_31038 : Constant  Value=-1
  Constant_-1_7c0cd : Constant  Value=-1
  Constant_-1_bfdba : Constant  Value=-1
  Constant_-1_eeca2 : Constant  Value=-1
  Constant_2.0_36b53 : Constant  Value=2.0
  Constant_2.0_38dac : Constant  Value=2.0
  Constant_2.0_774b7 : Constant  Value=2.0
  Constant_2.0_ff3e3 : Constant  Value=2.0
  Constant_K_A_11710 : Constant  Value=K_A
  Constant_K_A_7442c : Constant  Value=K_A
  Constant_K_A_f202f : Constant  Value=K_A
  Constant_K_F_3619e : Constant  Value=K_F
  Constant_K_s_574d1 : Constant  Value=K_s
  Constant_R_a_29e0d : Constant  Value=R_a
  Constant_R_a_3f5fe : Constant  Value=R_a
  Constant_T_A_f3abf : Constant  Value=T_A
  Constant_T_F_ea861 : Constant  Value=T_F
  Constant_V_ref_ff2f0 : Constant  Value=V_ref
  Constant_f0_3ca80 : Constant  Value=f0
  Constant_f0_4f5d9 : Constant  Value=f0
  Constant_pi_5bdeb : Constant  Value=pi
  Constant_pi_df3dc : Constant  Value=pi
  Constant_x_dd_869a6 : Constant  Value=x_dd
  Constant_x_dd_87abe : Constant  Value=x_dd
  Constant_x_dd_e9613 : Constant  Value=x_dd
  Constant_x_ddd_306fd : Constant  Value=x_ddd
  Constant_x_ddd_38dc9 : Constant  Value=x_ddd
  Constant_x_ddd_fe882 : Constant  Value=x_ddd
  Constant_x_l_0abc2 : Constant  Value=x_l
  Constant_x_l_3ea6d : Constant  Value=x_l
  Constant_x_l_978c9 : Constant  Value=x_l
  Constant_x_l_cd126 : Constant  Value=x_l
  Constant_x_l_e1d5e : Constant  Value=x_l
  Constant_x_l_f1050 : Constant  Value=x_l
  Constant_x_qd_61373 : Constant  Value=x_qd
  Constant_x_qd_73c9d : Constant  Value=x_qd
  Constant_x_qd_9e832 : Constant  Value=x_qd
  Constant_x_qdd_a2212 : Constant  Value=x_qdd
  Constant_x_qdd_df2e9 : Constant  Value=x_qdd
  Constant_x_qdd_df4b1 : Constant  Value=x_qdd
  Divide_2c2ae : Product  Inputs=*/
  Divide_36f01 : Product  Inputs=*/
  Divide_38c51 : Product  Inputs=*/
  Divide_59db1 : Product  Inputs=*/
  Divide_5fd17 : Product  Inputs=*/
  Divide_94042 : Product  Inputs=*/
  Divide_96028 : Product  Inputs=*/
  Divide_d2b4c : Product  Inputs=*/
  Divide_d8b0a : Product  Inputs=*/
  Divide_e79d2 : Product  Inputs=*/
  MathFunc_sqrt_83093 : Sqrt
  Power_2389f : Math  Operator=pow
  Power_fcd26 : Math  Operator=pow
  Product_00f9d : Product
  Product_0e948 : Product
  Product_15a68 : Product
  Product_25242 : Product
  Product_27ce4 : Product
  Product_3bb11 : Product
  Product_3d77d : Product
  Product_422bb : Product
  Product_4e670 : Product
  Product_52d4e : Product
  Product_55f3e : Product
  Product_5ccbd : Product
  Product_70f75 : Product
  Product_74801 : Product
  Product_75b81 : Product
  Product_8c408 : Product
  Product_91555 : Product
  Product_9391a : Product
  Product_ab62e : Product
  Product_c924d : Product
  Product_dff5c : Product
  Product_f28da : Product
  Product_f382d : Product
  Subtract_05fec : Sum  Inputs=+-
  Subtract_18cf7 : Sum  Inputs=+-
  Subtract_2b013 : Sum  Inputs=+-
  Subtract_46992 : Sum  Inputs=+-
  Subtract_93dc5 : Sum  Inputs=+-
  Subtract_ba6cb : Sum  Inputs=+-
  Subtract_da76f : Sum  Inputs=+-
  Subtract_dd4a3 : Sum  Inputs=+-
  Subtract_f0d62 : Sum  Inputs=+-
  Blockout_d_V_f_SG_D_2_ff4c4 : Outport
  wires:
  Constant_-1_eeca2/1 -> Product_ab62e/1
  Constant_2.0_ff3e3/1 -> Product_52d4e/1
  Constant_-1_31038/1 -> Product_4e670/1
  Product_52d4e/1 -> Product_91555/1
  Product_4e670/1 -> Add_398c1/1
  Constant_x_l_f1050/1 -> Product_0e948/2
  Constant_x_l_e1d5e/1 -> Product_4e670/2
  State_psi_1d_SG_D_2_6ad6a/1 -> Product_ab62e/2
  Constant_x_l_0abc2/1 -> Subtract_2b013/2
  Constant_x_dd_869a6/1 -> Subtract_da76f/1
  Product_c924d/1 -> Divide_d2b4c/1
  Constant_x_ddd_306fd/1 -> Subtract_da76f/2
  Constant_x_qd_61373/1 -> Add_bbddb/2
  Add_398c1/1 -> Product_f28da/2
  Constant_x_qdd_a2212/1 -> Add_398c1/2
  Constant_-1_18504/1 -> Product_27ce4/1
  Constant_x_dd_e9613/1 -> Subtract_2b013/1
  Subtract_ba6cb/1 -> Add_fd2ac/1
  Power_fcd26/1 -> Add_4f9e1/1
  Constant_x_l_cd126/1 -> Product_27ce4/2
  Constant_2.0_36b53/1 -> Product_f382d/1
  Constant_x_qd_73c9d/1 -> Subtract_46992/1
  Constant_pi_5bdeb/1 -> Product_f382d/2
  Subtract_dd4a3/1 -> Product_5ccbd/2
  Constant_x_qdd_df4b1/1 -> Subtract_46992/2
  State_psi_fd_SG_D_2_2a738/1 -> Product_25242/1
  Constant_-1_1eeb1/1 -> Product_0e948/1
  Product_ab62e/1 -> Product_00f9d/1
  State_w_SG_D_2_e6aa6/1 -> Product_70f75/2
  Subtract_da76f/1 -> Product_00f9d/2
  Constant_x_dd_87abe/1 -> Subtract_f0d62/1
  State_psi_q_SG_D_2_14190/1 -> Add_fd2ac/2
  State_w_SG_D_2_40010/1 -> Product_15a68/2
  Subtract_93dc5/1 -> Product_25242/2
  Constant_x_l_3ea6d/1 -> Subtract_f0d62/2
  Add_19da6/1 -> Add_2842c/1
  Constant_x_ddd_fe882/1 -> Subtract_93dc5/1
  Constant_x_l_978c9/1 -> Subtract_93dc5/2
  State_psi_gq_SG_D_2_0beb3/1 -> Product_f28da/1
  Product_27ce4/1 -> Add_d3ce1/1
  Subtract_2b013/1 -> Divide_59db1/2
  Constant_x_qd_9e832/1 -> Add_d3ce1/2
  Product_15a68/1 -> Divide_d8b0a/1
  State_psi_kq_SG_D_2_49fef/1 -> Product_3bb11/1
  Subtract_46992/1 -> Product_3bb11/2
  Product_25242/1 -> Divide_59db1/1
  State_V_f_SG_D_2_79586/1 -> Subtract_18cf7/2
  Product_0e948/1 -> Add_bbddb/1
  Product_00f9d/1 -> Divide_94042/1
  Divide_36f01/1 -> Subtract_ba6cb/1
  Subtract_f0d62/1 -> Divide_94042/2
  Product_f28da/1 -> Divide_36f01/1
  Add_d3ce1/1 -> Divide_36f01/2
  Product_3bb11/1 -> Divide_e79d2/1
  Divide_59db1/1 -> Subtract_dd4a3/2
  Constant_f0_4f5d9/1 -> Product_91555/2
  Add_bbddb/1 -> Divide_e79d2/2
  Divide_94042/1 -> Add_5abf2/1
  State_psi_d_SG_D_2_02653/1 -> Add_5abf2/2
  Divide_e79d2/1 -> Subtract_ba6cb/2
  Constant_-1_bfdba/1 -> Product_9391a/1
  Constant_R_a_3f5fe/1 -> Product_9391a/2
  Constant_f0_3ca80/1 -> Product_3d77d/2
  Add_5abf2/1 -> Subtract_dd4a3/1
  Product_9391a/1 -> Product_5ccbd/1
  Constant_pi_df3dc/1 -> Product_52d4e/2
  State_psi_q_SG_D_2_06b5a/1 -> Product_15a68/1
  Constant_R_a_29e0d/1 -> Product_c924d/1
  State_E_fd_SG_D_2_d52e1/1 -> Product_74801/2
  Add_fd2ac/1 -> Product_c924d/2
  State_psi_d_SG_D_2_55d30/1 -> Product_70f75/1
  Product_f382d/1 -> Product_3d77d/1
  Product_5ccbd/1 -> Divide_96028/1
  Constant_x_ddd_38dc9/1 -> Divide_96028/2
  Product_91555/1 -> Divide_d8b0a/2
  Constant_x_qdd_df2e9/1 -> Divide_d2b4c/2
  Product_70f75/1 -> Divide_2c2ae/1
  Product_3d77d/1 -> Divide_2c2ae/2
  Divide_96028/1 -> Add_59e32/1
  Divide_d8b0a/1 -> Add_59e32/2
  Divide_d2b4c/1 -> Add_1f75a/1
  Divide_2c2ae/1 -> Add_1f75a/2
  Constant_-1_7c0cd/1 -> Product_74801/1
  Add_59e32/1 -> Power_fcd26/1
  Constant_2.0_38dac/1 -> Power_fcd26/2
  Add_1f75a/1 -> Power_2389f/1
  Constant_2.0_774b7/1 -> Power_2389f/2
  Product_74801/1 -> Product_422bb/1
  Constant_K_A_7442c/1 -> Product_422bb/2
  Constant_K_s_574d1/1 -> Product_dff5c/1
  State_Px_3_SG_D_2_61526/1 -> Product_dff5c/2
  Power_2389f/1 -> Add_4f9e1/2
  Product_422bb/1 -> Product_8c408/1
  Constant_K_F_3619e/1 -> Product_8c408/2
  Product_dff5c/1 -> Add_d1505/1
  Constant_V_ref_ff2f0/1 -> Add_d1505/2
  Add_4f9e1/1 -> MathFunc_sqrt_83093/1
  Product_8c408/1 -> Divide_38c51/1
  Constant_T_F_ea861/1 -> Divide_38c51/2
  Constant_K_A_f202f/1 -> Product_55f3e/1
  State_R_f_SG_D_2_4eb2e/1 -> Product_55f3e/2
  Add_d1505/1 -> Subtract_05fec/1
  MathFunc_sqrt_83093/1 -> Subtract_05fec/2
  Divide_38c51/1 -> Add_19da6/1
  Product_55f3e/1 -> Add_19da6/2
  Constant_K_A_11710/1 -> Product_75b81/1
  Subtract_05fec/1 -> Product_75b81/2
  Product_75b81/1 -> Add_2842c/2
  Add_2842c/1 -> Subtract_18cf7/1
  Subtract_18cf7/1 -> Divide_5fd17/1
  Constant_T_A_f3abf/1 -> Divide_5fd17/2
  Divide_5fd17/1 -> Blockout_d_V_f_SG_D_2_ff4c4/1

== system case8/SG_D_2/d_psi_1d_SG_D_2_block ==
  note: d_psi_1d_SG_D_2 in case8
      | $-\frac{\psi _{\mathrm{1d},\mathrm{SG},D,2}-\psi _{\mathrm{fd},\mathrm{SG},D,2}+\frac{\left(x_{\mathrm{dd}}-x_{l}\right)\,\left(\frac{\psi _{\mathrm{1d},\mathrm{SG},D,2}\,\left(x_{\mathrm{dd}}-x_{\mathrm{ddd}}\right)}{x_{\mathrm{dd}}-x_{l}}-\psi _{d,\mathrm{SG},D,2}+\frac{\psi _{\mathrm{fd},\mathrm{SG},D,2}\,\left(x_{\mathrm{ddd}}-x_{l}\right)}{x_{\mathrm{dd}}-x_{l}}\right)}{x_{\mathrm{ddd}}}}{T_{\mathrm{ddd}}}$
      | Automatically generated on 2025-10-31 19:29:49 .
  State_psi_1d_SG_D_2_34802 : Inport
  State_psi_fd_SG_D_2_ceb12 : Inport  Port=2
  State_psi_1d_SG_D_2_f87fc : Inport  Port=3
  State_psi_d_SG_D_2_bd43f : Inport  Port=4
  State_psi_fd_SG_D_2_a1da1 : Inport  Port=5
  Add_02fd9 : Sum
  Add_58768 : Sum
  Add_caef2 : Sum
  Constant_-1_cc89f : Constant  Value=-1
  Constant_-1_de763 : Constant  Value=-1
  Constant_T_ddd_2034a : Constant  Value=T_ddd
  Constant_x_dd_0b947 : Constant  Value=x_dd
  Constant_x_dd_658ff : Constant  Value=x_dd
  Constant_x_dd_6b4c2 : Constant  Value=x_dd
  Constant_x_dd_def58 : Constant  Value=x_dd
  Constant_x_ddd_562a6 : Constant  Value=x_ddd
  Constant_x_ddd_5a3ac : Constant  Value=x_ddd
  Constant_x_ddd_97772 : Constant  Value=x_ddd
  Constant_x_l_1f432 : Constant  Value=x_l
  Constant_x_l_3d73c : Constant  Value=x_l
  Constant_x_l_79b40 : Constant  Value=x_l
  Constant_x_l_96b43 : Constant  Value=x_l
  Divide_56795 : Product  Inputs=*/
  Divide_84823 : Product  Inputs=*/
  Divide_b80b9 : Product  Inputs=*/
  Divide_be9cb : Product  Inputs=*/
  Product_22e0e : Product
  Product_53626 : Product
  Product_626ee : Product
  Product_6ef09 : Product
  Product_d49a0 : Product
  Subtract_0f8c3 : Sum  Inputs=+-
  Subtract_2f66b : Sum  Inputs=+-
  Subtract_62adb : Sum  Inputs=+-
  Subtract_9b5c5 : Sum  Inputs=+-
  Subtract_a35ae : Sum  Inputs=+-
  Subtract_b153c : Sum  Inputs=+-
  Blockout_d_psi_1d_SG_D_2_8d877 : Outport
  wires:
  Subtract_62adb/1 -> Product_6ef09/2
  Constant_x_l_96b43/1 -> Subtract_9b5c5/2
  Divide_be9cb/1 -> Add_02fd9/2
  Subtract_a35ae/1 -> Product_22e0e/2
  Constant_-1_cc89f/1 -> Product_53626/1
  Constant_x_dd_0b947/1 -> Subtract_b153c/1
  Divide_b80b9/1 -> Blockout_d_psi_1d_SG_D_2_8d877/1
  State_psi_fd_SG_D_2_ceb12/1 -> Add_58768/2
  State_psi_1d_SG_D_2_f87fc/1 -> Product_53626/2
  Divide_56795/1 -> Subtract_a35ae/2
  Constant_x_ddd_97772/1 -> Subtract_b153c/2
  State_psi_1d_SG_D_2_34802/1 -> Product_626ee/2
  Product_53626/1 -> Product_d49a0/1
  Subtract_b153c/1 -> Product_d49a0/2
  Constant_x_dd_658ff/1 -> Subtract_9b5c5/1
  Constant_x_ddd_562a6/1 -> Subtract_62adb/1
  Constant_x_l_79b40/1 -> Subtract_62adb/2
  Product_d49a0/1 -> Divide_84823/1
  Subtract_9b5c5/1 -> Divide_84823/2
  State_psi_fd_SG_D_2_a1da1/1 -> Product_6ef09/1
  Constant_x_dd_def58/1 -> Subtract_2f66b/1
  Constant_x_l_3d73c/1 -> Subtract_0f8c3/2
  Constant_x_l_1f432/1 -> Subtract_2f66b/2
  Constant_x_ddd_5a3ac/1 -> Divide_be9cb/2
  Divide_84823/1 -> Add_caef2/1
  State_psi_d_SG_D_2_bd43f/1 -> Add_caef2/2
  Product_6ef09/1 -> Divide_56795/1
  Subtract_2f66b/1 -> Divide_56795/2
  Constant_x_dd_6b4c2/1 -> Subtract_0f8c3/1
  Add_caef2/1 -> Subtract_a35ae/1
  Constant_-1_de763/1 -> Product_626ee/1
  Subtract_0f8c3/1 -> Product_22e0e/1
  Product_626ee/1 -> Add_58768/1
  Product_22e0e/1 -> Divide_be9cb/1
  Add_58768/1 -> Add_02fd9/1
  Add_02fd9/1 -> Divide_b80b9/1
  Constant_T_ddd_2034a/1 -> Divide_b80b9/2
